simulink model "sampleModel1980"  (R2023a)
settings: Solver=VariableStepAuto  StartTime=0.0  StopTime=10.0  RelTol=1e-3
libraries: hdlsllib x7, simulink x4
settings Model: Creator=user1  LastModifiedBy=user1

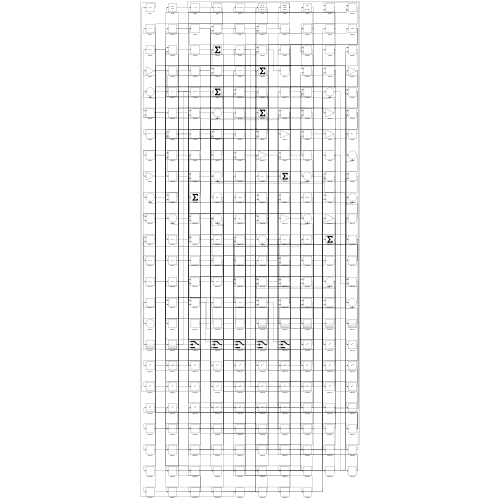
[thumbnail: Simulink's stored preview of the top-level diagram]
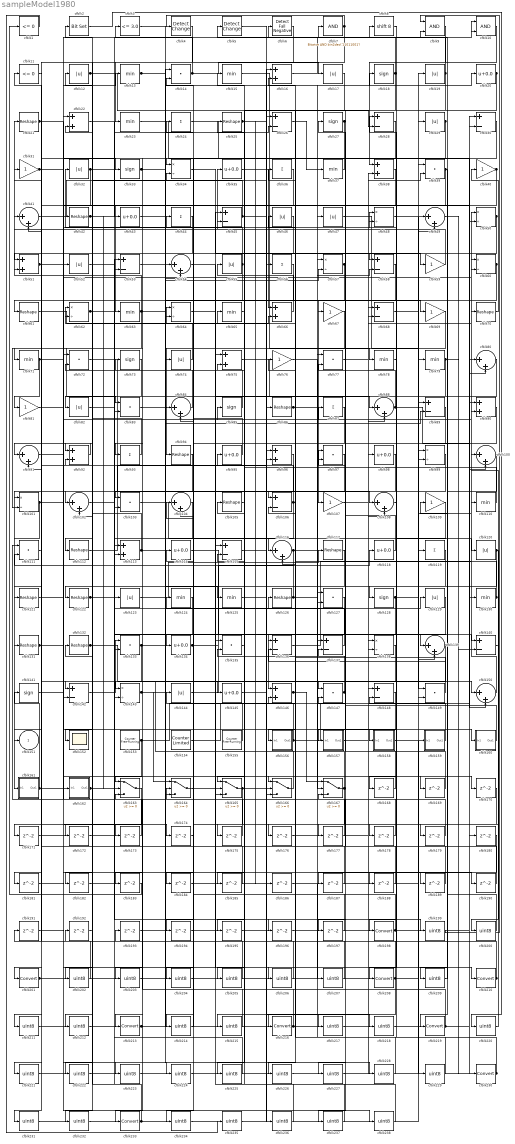
== system sampleModel1980 ==
  cfblk1 : hdlsllib/Logic and Bit Operations/Compare To Zero  relop=<=  OutDataTypeStr=boolean
  cfblk10 : Logic  AllPortsSameDT=off  OutDataTypeStr=boolean
  cfblk{41,49,54,80,84,88,91,100,102,104,108,116,139,150} (14 alike) : Sum  Inputs=|++
  cfblk{34,48,50,57,60,62,64,99,101,138,143} (11 alike) : Product  Inputs=*/  RndMeth=Zero  SaturateOnIntegerOverflow=on
  cfblk{14,39,72,77,83,97,103,111,127,133,135,147,149} (13 alike) : DotProduct  OutDataTypeStr=Inherit: Inherit via internal rule
  cfblk{21,25,42,61,70,86,94,105,112,117,121..122,126,131..132} (15 alike) : Reshape
  cfblk{26,28,30,45,53,58,68,89,106,115,136..137,140,142,148} (15 alike) : Sum  Inputs=+-
  cfblk{31,40,59,67,69,76,81,107,109} (9 alike) : Gain
  cfblk11 : hdlsllib/Logic and Bit Operations/Compare To Zero  relop=<=  OutDataTypeStr=boolean
  cfblk{13,15,23,37,63,65,71,78..79,110,124..125,130} (13 alike) : MinMax
  cfblk{16,22,38,51,66,75,90,92,96,113,146} (11 alike) : Sum
  cfblk{20,35,43,95,98,114,118,134,145} (9 alike) : Bias  Bias=0.0  SaturateOnIntegerOverflow=off
  cfblk{24,36,44,56,87,93,119} (7 alike) : Sum  Inputs=+
  cfblk{12,17,19,29,32,46..47,52,55,74,82,120,123,129,144} (15 alike) : Abs  SaturateOnIntegerOverflow=off
  cfblk{18,27,33,73,85,128,141} (7 alike) : Signum
  cfblk152 : Scope
  cfblk153 : hdlsllib/Sources/Counter Free-Running  NumBits=16  tsamp=-1
  cfblk154 : hdlsllib/Sources/Counter Limited  uplimit=7  tsamp=-1
  cfblk155 : hdlsllib/Sources/Counter Free-Running  NumBits=16  tsamp=-1
  cfblk156 : Subsystem
      settings: LibrarySourceBlock=|
      | hdlsllib/Ports &
      | Subsystems/Subsystem
  cfblk157 : Subsystem
      settings: LibrarySourceBlock=|
      | hdlsllib/Ports &
      | Subsystems/Subsystem
  cfblk158 : Subsystem
      settings: LibrarySourceBlock=|
      | hdlsllib/Ports &
      | Subsystems/Subsystem
  cfblk159 : Subsystem
      settings: LibrarySourceBlock=|
      | hdlsllib/Ports &
      | Subsystems/Subsystem
  cfblk160 : Subsystem
      settings: LibrarySourceBlock=|
      | hdlsllib/Ports &
      | Subsystems/Subsystem
  cfblk161 : Subsystem
      settings: LibrarySourceBlock=|
      | hdlsllib/Ports &
      | Subsystems/Subsystem
  cfblk162 : Subsystem
      settings: LibrarySourceBlock=|
      | hdlsllib/Ports &
      | Subsystems/Subsystem
  cfblk{163..167} (5 alike) : Switch  SaturateOnIntegerOverflow=off  InputSameDT=off
  cfblk{168..197} (30 alike) : Delay  SampleTime=1
  cfblk{198,201,208,210,213,216,219,230,233} (9 alike) : DataTypeConversion  SaturateOnIntegerOverflow=off  RndMeth=Floor
  cfblk{199..200,202..207,209,211..212,214..215,217..218,220..229,231..232,234..238} (32 alike) : DataTypeConversion  OutDataTypeStr=uint8  SaturateOnIntegerOverflow=off  RndMeth=Floor
  cfblk2 : simulink/Logic and Bit Operations/Bit Set  iBit=0
      settings: LibrarySourceBlock=|
      | hdlsllib/Logic and Bit
      | Operations/Bit Set
  cfblk3 : hdlsllib/Logic and Bit Operations/Compare To Constant  relop=<=  const=3.0  OutDataTypeStr=boolean
  cfblk4 : simulink/Logic and Bit Operations/Detect Change  vinit=0  OutDataTypeStr=boolean
      settings: LibrarySourceBlock=|
      | hdlsllib/Logic and Bit
      | Operations/Detect
      | Change
  cfblk5 : simulink/Logic and Bit Operations/Detect Change  vinit=0  OutDataTypeStr=boolean
      settings: LibrarySourceBlock=|
      | hdlsllib/Logic and Bit
      | Operations/Detect
      | Change
  cfblk6 : hdlsllib/Logic and Bit Operations/Detect Fall Negative  vinit=0  OutDataTypeStr=boolean
  cfblk7 : simulink/Logic and Bit Operations/Bitwise Operator  logicop=AND  UseBitMask=on  BitMask=bin2dec('11011001')  BitMaskRealWorld=Stored Integer
      settings: LibrarySourceBlock=|
      | hdlsllib/Logic and Bit
      | Operations/Bitwise
      | Operator
  cfblk8 : ArithShift  BitShiftNumber=8
  cfblk9 : Logic  AllPortsSameDT=off  OutDataTypeStr=boolean
  cfblk151 : Outport  VectorParamsAs1DForOutWhenUnconnected=off
  wires:
  cfblk59/1 -> cfblk35/1
  cfblk63/1 -> cfblk21/1, cfblk166/2, cfblk101/2
  cfblk10/1 -> cfblk38/1
  cfblk143/1 -> cfblk164/1, cfblk57/2
  cfblk72/1 -> cfblk108/1
  cfblk123/1 -> cfblk117/1
  cfblk57/1 -> cfblk83/1, cfblk71/1, cfblk187/1
  cfblk20/1 -> cfblk67/1, cfblk157/1(In1), cfblk177/1
  cfblk103/1 -> cfblk116/1
  cfblk133/1 -> cfblk89/2, cfblk211/1, cfblk212/1
  cfblk79/1 -> cfblk140/2, cfblk178/1
  cfblk58/1 -> cfblk107/1
  cfblk15/1 -> cfblk78/1
  cfblk26/1 -> cfblk37/1
  cfblk144/1 -> cfblk118/1
  cfblk29/1 -> cfblk93/1, cfblk182/1
  cfblk50/1 -> cfblk171/1, cfblk172/1
  cfblk116/1 -> cfblk111/2, cfblk170/1
  cfblk121/1 -> cfblk52/1
  cfblk35/1 -> cfblk66/1
  cfblk83/1 -> cfblk94/1
  cfblk56/1 -> cfblk61/1
  cfblk85/1 -> cfblk72/2
  cfblk78/1 -> cfblk164/2
  cfblk114/1 -> cfblk139/1
  cfblk36/1 -> cfblk82/1
  cfblk84/1 -> cfblk73/1
  cfblk104/1 -> cfblk213/1
  cfblk167/1 -> cfblk142/1, cfblk194/1
  cfblk53/1 -> cfblk125/1
  cfblk42/1 -> cfblk123/1, cfblk26/2, cfblk140/1
  cfblk159/1(Out1) -> cfblk28/1
  cfblk142/1 -> cfblk133/1
  cfblk4/1 -> cfblk23/1
  cfblk9/1 -> cfblk198/1
  cfblk47/1 -> cfblk149/1
  cfblk120/1 -> cfblk122/1, cfblk200/1
  cfblk65/1 -> cfblk165/1
  cfblk150/1 -> cfblk50/1
  cfblk157/1(Out1) -> cfblk68/1
  cfblk12/1 -> cfblk28/2, cfblk8/1
  cfblk55/1 -> cfblk32/1, cfblk84/2, cfblk103/2
  cfblk136/1 -> cfblk60/1
  cfblk6/1 -> cfblk102/1
  cfblk101/1 -> cfblk161/1(In1), cfblk206/1
  cfblk137/1 -> cfblk44/1
  cfblk8/1 -> cfblk58/1
  cfblk14/1 -> cfblk17/1, cfblk3/1
  cfblk132/1 -> cfblk147/1, cfblk126/1
  cfblk54/1 -> cfblk210/1
  cfblk7/1 -> cfblk4/1, cfblk101/1
  cfblk46/1 -> cfblk92/1
  cfblk100/1 -> cfblk219/1
  cfblk147/1 -> cfblk95/1, cfblk16/2
  cfblk127/1 -> cfblk146/1
  cfblk164/1 -> cfblk90/2
  cfblk31/1 -> cfblk33/1, cfblk190/1
  cfblk11/1 -> cfblk201/1
  cfblk112/1 -> cfblk86/1
  cfblk3/1 -> cfblk69/1
  cfblk149/1 -> cfblk46/1
  cfblk37/1 -> cfblk34/1
  cfblk153/1 -> cfblk163/1, cfblk80/2
  cfblk16/1 -> cfblk10/1
  cfblk161/1(Out1) -> cfblk141/1, cfblk60/2
  cfblk81/1 -> cfblk13/1
  cfblk67/1 -> cfblk84/1
  cfblk130/1 -> cfblk41/1, cfblk106/2, cfblk62/2
  cfblk106/1 -> cfblk116/2, cfblk51/2, cfblk113/2
  cfblk98/1 -> cfblk131/1
  cfblk131/1 -> cfblk160/1(In1), cfblk223/1
  cfblk155/1 -> cfblk114/1
  cfblk38/1 -> cfblk63/1
  cfblk77/1 -> cfblk39/2
  cfblk88/1 -> cfblk27/1, cfblk130/1
  cfblk22/1 -> cfblk165/2
  cfblk162/1(Out1) -> cfblk129/1, cfblk43/1
  cfblk49/1 -> cfblk230/1
  cfblk113/1 -> cfblk45/2, cfblk12/1
  cfblk165/1 -> cfblk169/1, cfblk204/1
  cfblk69/1 -> cfblk74/1
  cfblk74/1 -> cfblk62/1
  cfblk70/1 -> cfblk40/1
  cfblk18/1 -> cfblk5/1, cfblk145/1
  cfblk122/1 -> cfblk65/1, cfblk166/1
  cfblk145/1 -> cfblk26/1
  cfblk76/1 -> cfblk137/1
  cfblk94/1 -> cfblk103/1
  cfblk108/1 -> cfblk128/1
  cfblk32/1 -> cfblk7/1, cfblk142/2
  cfblk99/1 -> cfblk216/1
  cfblk62/1 -> cfblk165/3, cfblk106/1
  cfblk34/1 -> cfblk59/1
  cfblk93/1 -> cfblk2/1
  cfblk82/1 -> cfblk113/1
  cfblk41/1 -> cfblk16/1
  cfblk146/1 -> cfblk36/1, cfblk167/1
  cfblk19/1 -> cfblk6/1, cfblk156/1(In1)
  cfblk5/1 -> cfblk150/1
  cfblk109/1 -> cfblk208/1
  cfblk107/1 -> cfblk70/1
  cfblk160/1(Out1) -> cfblk137/2
  cfblk27/1 -> cfblk133/2, cfblk231/1
  cfblk45/1 -> cfblk22/2, cfblk120/1, cfblk195/1
  cfblk141/1 -> cfblk87/1
  cfblk61/1 -> cfblk66/2
  cfblk111/1 -> cfblk41/2
  cfblk48/1 -> cfblk139/2
  cfblk75/1 -> cfblk127/1
  cfblk134/1 -> cfblk68/2, cfblk24/1
  cfblk95/1 -> cfblk64/1
  cfblk154/1 -> cfblk56/1
  cfblk102/1 -> cfblk85/1
  cfblk60/1 -> cfblk152/1, cfblk112/1
  cfblk21/1 -> cfblk50/2, cfblk51/1, cfblk166/3
  cfblk126/1 -> cfblk102/2, cfblk58/2
  cfblk51/1 -> cfblk162/1(In1), cfblk174/1
  cfblk39/1 -> cfblk197/1, cfblk209/1, cfblk221/1
  cfblk25/1 -> cfblk186/1, cfblk199/1
  cfblk86/1 -> cfblk20/1, cfblk176/1
  cfblk105/1 -> cfblk15/1
  cfblk68/1 -> cfblk79/1
  cfblk128/1 -> cfblk110/1, cfblk143/2
  cfblk13/1 -> cfblk167/2, cfblk188/1
  cfblk156/1(Out1) -> cfblk34/2, cfblk89/1
  cfblk96/1 -> cfblk233/1
  cfblk40/1 -> cfblk136/1, cfblk121/1
  cfblk64/1 -> cfblk88/1
  cfblk118/1 -> cfblk97/1
  cfblk23/1 -> cfblk80/1
  cfblk166/1 -> cfblk105/1
  cfblk110/1 -> cfblk75/2
  cfblk30/1 -> cfblk151/1
  cfblk80/1 -> cfblk143/1
  cfblk24/1 -> cfblk150/2
  cfblk28/1 -> cfblk134/1
  cfblk139/1 -> cfblk136/2, cfblk237/1
  cfblk71/1 -> cfblk158/1(In1), cfblk10/2, cfblk81/1
  cfblk66/1 -> cfblk25/1
  cfblk92/1 -> cfblk91/1
  cfblk33/1 -> cfblk18/1, cfblk189/1
  cfblk91/1 -> cfblk48/1
  cfblk90/1 -> cfblk168/1
  cfblk168/1 -> cfblk77/2
  cfblk169/1 -> cfblk147/2
  cfblk171/1 -> cfblk83/2
  cfblk129/1 -> cfblk173/1
  cfblk173/1 -> cfblk22/1
  cfblk174/1 -> cfblk14/2
  cfblk87/1 -> cfblk175/1
  cfblk175/1 -> cfblk111/1
  cfblk176/1 -> cfblk38/2
  cfblk177/1 -> cfblk72/1
  cfblk178/1 -> cfblk45/1
  cfblk140/1 -> cfblk179/1
  cfblk179/1 -> cfblk57/1
  cfblk163/1 -> cfblk181/1
  cfblk182/1 -> cfblk53/2
  cfblk44/1 -> cfblk183/1
  cfblk183/1 -> cfblk1/1
  cfblk117/1 -> cfblk184/1
  cfblk184/1 -> cfblk149/2
  cfblk97/1 -> cfblk185/1
  cfblk185/1 -> cfblk75/1
  cfblk187/1 -> cfblk91/2
  cfblk188/1 -> cfblk146/2
  cfblk189/1 -> cfblk48/2
  cfblk190/1 -> cfblk167/3
  cfblk192/1 -> cfblk92/2
  cfblk193/1 -> cfblk108/2
  cfblk194/1 -> cfblk127/2
  cfblk195/1 -> cfblk88/2
  cfblk52/1 -> cfblk196/1
  cfblk196/1 -> cfblk39/1
  cfblk197/1 -> cfblk64/2
  cfblk198/1 -> cfblk30/2, cfblk144/1
  cfblk199/1 -> cfblk9/1
  cfblk200/1 -> cfblk9/2
  cfblk201/1 -> cfblk98/1, cfblk159/1(In1)
  cfblk73/1 -> cfblk202/1
  cfblk202/1 -> cfblk11/1
  cfblk124/1 -> cfblk203/1
  cfblk203/1 -> cfblk47/1
  cfblk204/1 -> cfblk124/1
  cfblk135/1 -> cfblk205/1
  cfblk205/1 -> cfblk42/1
  cfblk206/1 -> cfblk135/1
  cfblk186/1 -> cfblk207/1
  cfblk207/1 -> cfblk135/2
  cfblk208/1 -> cfblk14/1, cfblk215/1
  cfblk209/1 -> cfblk109/1
  cfblk210/1 -> cfblk193/1, cfblk192/1, cfblk191/1, cfblk31/1
  cfblk211/1 -> cfblk54/1
  cfblk212/1 -> cfblk54/2
  cfblk213/1 -> cfblk97/2, cfblk30/1
  cfblk89/1 -> cfblk214/1
  cfblk214/1 -> cfblk104/1
  cfblk215/1 -> cfblk104/2
  cfblk216/1 -> cfblk19/1, cfblk164/3
  cfblk180/1 -> cfblk217/1
  cfblk217/1 -> cfblk99/1
  cfblk125/1 -> cfblk218/1
  cfblk218/1 -> cfblk99/2
  cfblk219/1 -> cfblk180/1, cfblk163/3
  cfblk2/1 -> cfblk220/1
  cfblk220/1 -> cfblk100/1
  cfblk221/1 -> cfblk100/2
  cfblk138/1 -> cfblk222/1
  cfblk222/1 -> cfblk29/1
  cfblk223/1 -> cfblk138/1
  cfblk181/1 -> cfblk224/1
  cfblk224/1 -> cfblk138/2
  cfblk119/1 -> cfblk225/1
  cfblk225/1 -> cfblk53/1
  cfblk17/1 -> cfblk226/1
  cfblk226/1 -> cfblk119/1
  cfblk148/1 -> cfblk227/1
  cfblk227/1 -> cfblk90/1
  cfblk43/1 -> cfblk228/1
  cfblk228/1 -> cfblk148/1
  cfblk158/1(Out1) -> cfblk229/1
  cfblk229/1 -> cfblk148/2
  cfblk230/1 -> cfblk76/1, cfblk77/1
  cfblk231/1 -> cfblk49/1
  cfblk172/1 -> cfblk232/1
  cfblk232/1 -> cfblk49/2
  cfblk233/1 -> cfblk163/2, cfblk132/1
  cfblk170/1 -> cfblk234/1
  cfblk234/1 -> cfblk96/1
  cfblk1/1 -> cfblk235/1
  cfblk235/1 -> cfblk96/2
  cfblk115/1 -> cfblk236/1
  cfblk236/1 -> cfblk55/1
  cfblk237/1 -> cfblk115/1
  cfblk191/1 -> cfblk238/1
  cfblk238/1 -> cfblk115/2

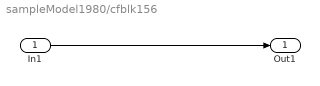
== system sampleModel1980/cfblk156 ==
  In1 : Inport
  Out1 : Outport
  wires:
  In1/1 -> Out1/1

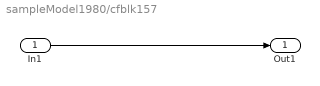
== system sampleModel1980/cfblk157 ==
  In1 : Inport
  Out1 : Outport
  wires:
  In1/1 -> Out1/1

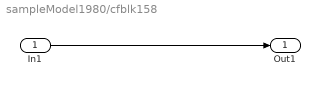
== system sampleModel1980/cfblk158 ==
  In1 : Inport
  Out1 : Outport
  wires:
  In1/1 -> Out1/1

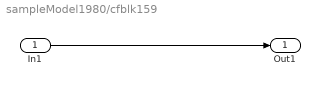
== system sampleModel1980/cfblk159 ==
  In1 : Inport
  Out1 : Outport
  wires:
  In1/1 -> Out1/1

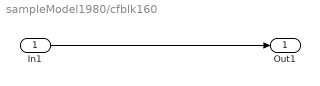
== system sampleModel1980/cfblk160 ==
  In1 : Inport
  Out1 : Outport
  wires:
  In1/1 -> Out1/1

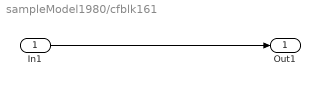
== system sampleModel1980/cfblk161 ==
  In1 : Inport
  Out1 : Outport
  wires:
  In1/1 -> Out1/1

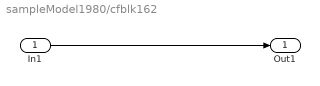
== system sampleModel1980/cfblk162 ==
  In1 : Inport
  Out1 : Outport
  wires:
  In1/1 -> Out1/1
